simulink model "FMECUService"  (R2024a)
settings: Solver=VariableStepAuto  StartTime=0.0  StopTime=inf  RelTol=1e-3
libraries: sldrtlib x1
settings Model: Creator=ABDERRAZEK  LastModifiedBy=ABDERRAZEK

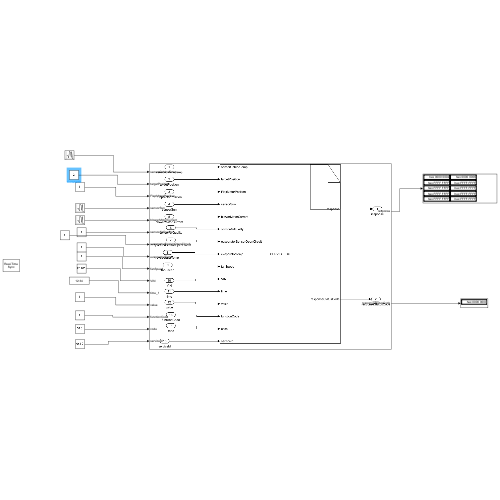
[thumbnail: Simulink's stored preview of the top-level diagram]
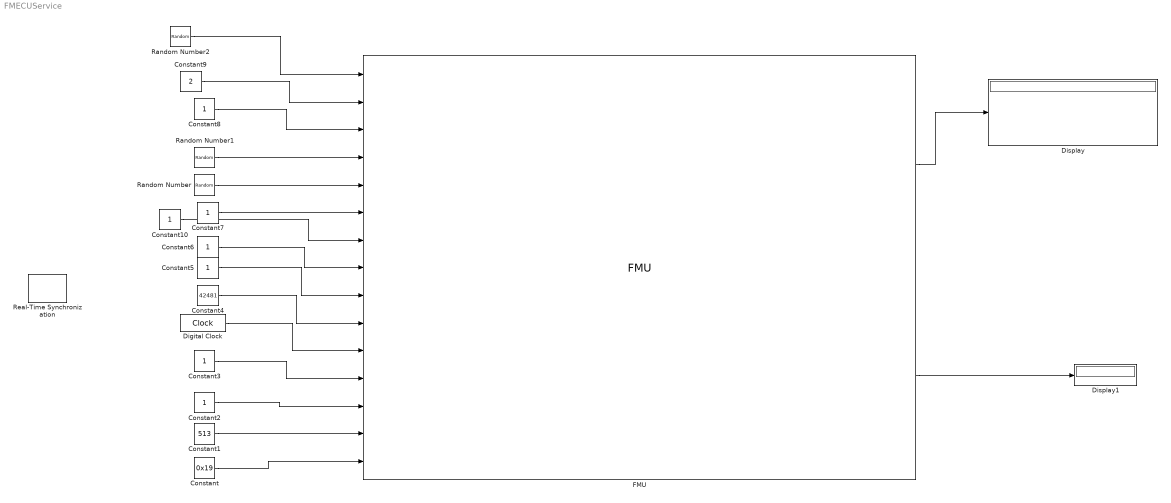
== system FMECUService ==
  Constant : Constant  Value=0x19  OutDataTypeStr=int32
  Constant1 : Constant  Value=513  OutDataTypeStr=int32
  Constant10 : Constant  OutDataTypeStr=int32
  Constant2 : Constant  OutDataTypeStr=int32
  Constant3 : Constant  OutDataTypeStr=double
  Constant4 : Constant  Value=42481  OutDataTypeStr=int32
  Constant{5..8} (4 alike) : Constant
  Constant9 : Constant  Value=2
  Digital Clock : DigitalClock
  Display : Display
      settings: Format=hex (Stored Integer)
  Display1 : Display
      settings: Format=hex (Stored Integer)
  FMU : FMU  FMUName=SERVICEECUsimlik.fmu  FMUMode=CoSimulation  FMUCreateBusObject=off  FMUInitializeEnumObject=off
      mask Type: SERVICEECUsimlik [Co-Simulation, v2.0]
      mask Display:
      | if (exist([Simulink.fileGenControl('get','CacheFolder') '\slprj\_fmu\55045776cb6cc7ffa340d3ded4d99871\SERVICEECUsimlik\model.png'],'file'))
      |     image([Simulink.fileGenControl('get','CacheFolder') '\slprj\_fmu\55045776cb6cc7ffa340d3ded4d99871\SERVICEECUsimlik\model.png']);
      | else
      |     disp('SERVICEECUsimlik');
      | end
      | port_label('output',1,'response');
      | port_label('output',2,'responseStatusCode');
      | port_label('input',1,'sensorCabineTemp');
      | port_label('input',2,'targetPosition');
      | port_label('input',3,'FlapMotorPosition');
      | port_label('input',4,'sensorSun');
      | port_label('input',5,'blowerMotorCurrent');
      | port_label('input',6,'sensorAirQuality');
      | port_label('input',7,'evaporatorSensorOpenCircuit');
      | port_label('input',8,'evaporatorTemp');
      | port_label('input',9,'fanSpeed');
      | port_label('input',10,'VIN');
      | port_label('input',11,'time_1');
      | port_label('input',12,'value');
      | port_label('input',13,'functionCode');
      | port_label('input',14,'code');
      | port_label('input',15,'serviceId');
  Random Number : RandomNumber  Variance=10  SampleTime=0.1
  Random Number1 : RandomNumber  Variance=100  SampleTime=1
  Random Number2 : RandomNumber  Variance=100  SampleTime=15
  Real-Time Synchronization : sldrtlib/Real-Time Synchronization  SampleTime=0.2  MaxMissedTicks=10  ShowMissedTicks=off  YieldWhenWaiting=on
  wires:
  FMU/1 -> Display/1
  FMU/2 -> Display1/1
  Constant/1 -> FMU/15
  Constant1/1 -> FMU/14
  Constant2/1 -> FMU/13
  Constant3/1 -> FMU/12
  Digital Clock/1 -> FMU/11
  Constant4/1 -> FMU/10
  Constant5/1 -> FMU/9
  Constant6/1 -> FMU/8
  Constant7/1 -> FMU/6
  Random Number/1 -> FMU/5
  Random Number1/1 -> FMU/4
  Constant8/1 -> FMU/3
  Constant9/1 -> FMU/2
  Random Number2/1 -> FMU/1
  Constant10/1 -> FMU/7
